simulink model "PistonEngineTestbed"  (R2026a)
settings: Solver=VariableStepAuto  StopTime=0.2  AbsTol=1e-3  EnableMultiTasking=on
libraries: fl_lib x18, nesl_utility x5, sdl_lib x3
CloseFcn:
  | try,close(h1_PistonEngineTestbed),end
  | clear h1_PistonEngineTestbed
  | 
  | 
  | clear simlog_PistonEngineTestbed
Description:
  | Piston Engine Testbed
settings Model: FPTRunName=Active  ExtModeAutoUpdateStatusClock=off  Creator=The MathWorks, Inc.  LastModifiedBy=The MathWorks, Inc.
settings SolverCC: ZcThreshold=0
settings DataIOCC: SignalLoggingName=logsout_PistonEngineTestbed
settings OptimizationCC: InitFltsAndDblsToZero=on  BufferReusableBoundary=off
settings DebuggingCC: SaveWithParameterizedLinksMsg=none  SignalResolutionControl=TryResolveAllWithWarning  MultiTaskDSMMsg=warning  MultiTaskCondExecSysMsg=none  SigSpecEnsureSampleTimeMsg=none  BusObjectLabelMismatch=none  PregeneratedLibrarySubsystemCodeDiagnostic=none
settings HardwareCC: ProdHWDeviceType=32-bit Generic  TargetBitPerPointer=64.0  TargetBitPerSizeT=64.0  TargetBitPerPtrDiffT=64.0  TargetLongLongMode=on  TargetIntDivRoundTo=Zero  TargetEndianess=LittleEndian  TargetWordSize=64.0  TargetHWDeviceType=MATLAB Host  ProdEqTarget=off
settings GRTTargetCC: CombineOutputUpdateFcns=off  GRTInterface=on
settings SimscapeCC: SimscapeNominalValues="[{\"value\":\"1\",\"unit\":\"A\"},{\"value\":\"1\",\"unit\":\"bar\"},{\"value\":\"1\",\"unit\":\"cm^2\"},{\"value\":\"1\",\"unit\":\"cm^3/s\"},{\"value\":\"1\",\"unit\":\"kJ/kg\"},{\"value\":\"1\",\"unit\":\"kW\"},{\"value\":\"1\",\"unit\":\"l\"},{\"value\":\"1\",\"unit\":\"N\"},{\"value\":\"1\",\"unit\":\"N*m\"},{\"value\":\"1\",\"unit\":\"V\"}]"  SimscapeLogSimulationStatistics=on  SimscapeLogName=simlog_PistonEngineTestbed  SimscapeLogDataHistory=5000.0

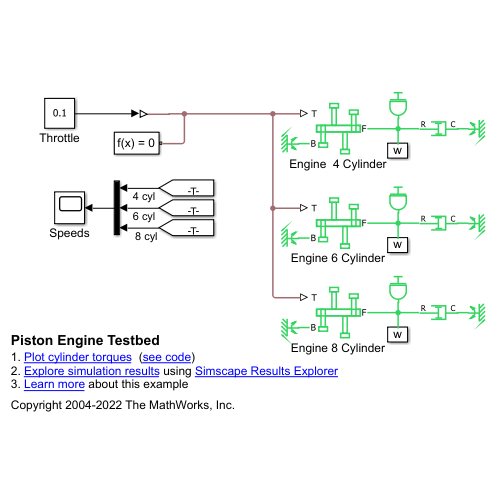
[thumbnail: Simulink's stored preview of the top-level diagram]
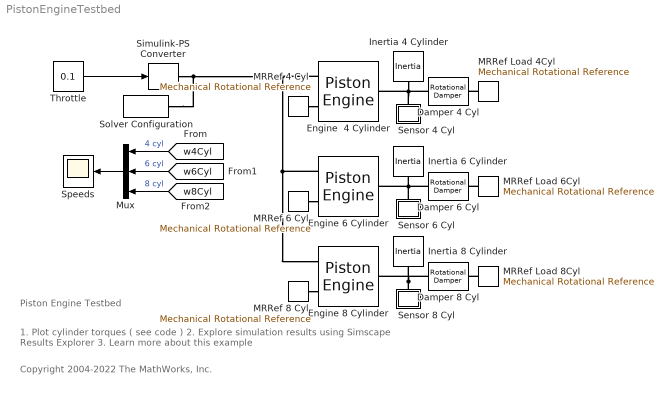
== system PistonEngineTestbed ==
  note: Piston Engine Testbed
  note: 1. Plot cylinder torques ( see code )
      | 2. Explore simulation results using Simscape Results Explorer
      | 3. Learn more about this example
  note: Copyright 2004-2022 The MathWorks, Inc.
  Damper 4 Cyl : fl_lib/Mechanical/Rotational Elements/Rotational Damper  D=0.0885 N*m/(rad/s)  w_specify=off  w_priority=None  w=0 rad/s  w_nominal_specify=off  w_nominal_value=1  w_nominal_unit=rad/s  t_specify=off  t_priority=None  t=0 N*m  t_nominal_specify=off  t_nominal_value=1  t_nominal_unit=N*m
  Damper 6 Cyl : fl_lib/Mechanical/Rotational Elements/Rotational Damper  D=0.0885 N*m/(rad/s)  w_specify=off  w_priority=None  w=0 rad/s  w_nominal_specify=off  w_nominal_value=1  w_nominal_unit=rad/s  t_specify=off  t_priority=None  t=0 N*m  t_nominal_specify=off  t_nominal_value=1  t_nominal_unit=N*m
  Damper 8 Cyl : fl_lib/Mechanical/Rotational Elements/Rotational Damper  D=0.0885 N*m/(rad/s)  w_specify=off  w_priority=None  w=0 rad/s  w_nominal_specify=off  w_nominal_value=1  w_nominal_unit=rad/s  t_specify=off  t_priority=None  t=0 N*m  t_nominal_specify=off  t_nominal_value=1  t_nominal_unit=N*m
  Engine  4 Cylinder : sdl_lib/Engines & Motors/Piston Engine  piston_num=4  theta_offset_vector=[0.0, 180.0, 360.0, -180.0] deg  bore=.10 m  stroke=.06 m  rod=.1 m  stroke_num=4  parameterization=1  angle_vector=[-360.0, -90.0, -30.0, 10.0, 30.0, 90.0, 160.0, 360.0] deg  throttle_vector=[0.0, 0.3, 0.8, 1.0]  velocity_vector=[0.0, 1000.0, 6000.0] rpm  pressure_vector=[0.0, 3.0, 20.0, 50.0, 20.0, 10.0, 8.0, 0.0] bar  pressure_matrix=[0.0, 0.0, 0.0, 0.0; 0.0, 0.9, 2.4, 3.0; 0.0, 6.0, 16.0, 20.0; 0.0, 15.0, 40.0, 50.0; 0.0, 6.0, 16.0, 20.0; 0.0, 3.0, 8.0, 10.0; 0.0, 2.4, 6.4, 8.0; 0.0, 0.0, 0.0, 0.0] bar  pressure_matrix_3D=cat(3, [0.0, 0.0, 0.0, 0.0; 0.0, 0.9, 2.4, 3.0; 0.0, 6.0, 16.0, 20.0; 0.0, 15.0, 40.0, 50.0; 0.0, 6.0, 16.0, 20.0; 0.0, 3.0, 8.0, 10.0; 0.0, 2.4, 6.4, 8.0; 0.0, 0.0, 0.0, 0.0], [0.0, 0.0, 0.0, 0.0; 0.0, 0.9, 2.4, 3.0; 0.0, 6.0, 16.0, 20.0; 0.0, 15.0, 40.0, 50.0; 0.0, 6.0, 16.0, 20.0; 0.0, 3.0, 8.0, 10.0; 0.0, 2.4, 6.4, 8.0; 0.0, 0.0, 0.0, 0.0], [0.0, 0.0, 0.0, 0.0; 0.0, 0.9, 2.4, 3.0; 0.0, 6.0, 16.0, 20.0; 0.0, 15.0, 40.0, 50.0; 0.0, 6.0, 16.0, 20.0; 0.0, 3.0, 8.0, 10.0; 0.0, 2.4, 6.4, 8.0; 0.0, 0.0, 0.0, 0.0]) bar  shaft_dynamics=0  stiffness=1e6 N*m/rad  damping=1000 N*m/(rad/s)  inertia=.02 kg*m^2  initial_deflection=0 deg  initial_velocity=0 rpm  mu_visc=[0.0, 0.01] N*m/(rad/s)  theta_init=0 deg  fc_model=sdl.enum.fuel_consumption_model.FuelOff  fc_per_rev=25 mg/rev  fc_w_tab=[1000, 2000, 3000, 4000, 5000, 6000] rpm  fc_trq_tab=[0, 80, 160, 200, 240, 320, 360, 400] N*m  fc_tab=[.5, .9, 1.4, 1.6, 1.9, 2.7, 3.4, 4.4; 1, 1.7, 2.7, 3.1, 3.6, 5, 6, 7.4; 1.4, 2.7, 4, 4.8, 5.6, 7.5, 8.5, 10.5; 2, 3.6, 5.8, 6.7, 8, 10.4, 11.7, 13.3; 2.5, 4.8, 7.9, 9.4, 10.8, 14, 16.2, 18.6; 3.1, 6, 10.3, 11.9, 13.8, 18.4, 22, 26.5] g/s  bmep_tab=[0, 250, 500, 625, 750, 1000, 1150, 1250] kPa  bsfc_tab=[410, 380, 300, 280, 270, 290, 320, 380; 410, 370, 290, 270, 260, 270, 285, 320; 415, 380, 290, 275, 265, 270, 270, 300; 420, 390, 310, 290, 285, 280, 280, 285; 430, 410, 340, 320, 310, 300, 310, 320; 450, 430, 370, 340, 330, 330, 350, 380] g/hr/kW  fc_interp_method=simscape.enum.interpolation.linear
  Engine 6 Cylinder : sdl_lib/Engines & Motors/Piston Engine  piston_num=6  theta_offset_vector=[0.0, 120.0, 240.0, 360.0, -240.0, -120.0] deg  bore=.10 m  stroke=.06 m  rod=.1 m  stroke_num=4  parameterization=1  angle_vector=[-360.0, -90.0, -30.0, 10.0, 30.0, 90.0, 160.0, 360.0] deg  throttle_vector=[0.0, 0.3, 0.8, 1.0]  velocity_vector=[0.0, 1000.0, 6000.0] rpm  pressure_vector=[0.0, 3.0, 20.0, 50.0, 20.0, 10.0, 8.0, 0.0]*4/6 bar  pressure_matrix=[0.0, 0.0, 0.0, 0.0; 0.0, 0.9, 2.4, 3.0; 0.0, 6.0, 16.0, 20.0; 0.0, 15.0, 40.0, 50.0; 0.0, 6.0, 16.0, 20.0; 0.0, 3.0, 8.0, 10.0; 0.0, 2.4, 6.4, 8.0; 0.0, 0.0, 0.0, 0.0]*4/6 bar  pressure_matrix_3D=cat(3, [0.0, 0.0, 0.0, 0.0; 0.0, 0.9, 2.4, 3.0; 0.0, 6.0, 16.0, 20.0; 0.0, 15.0, 40.0, 50.0; 0.0, 6.0, 16.0, 20.0; 0.0, 3.0, 8.0, 10.0; 0.0, 2.4, 6.4, 8.0; 0.0, 0.0, 0.0, 0.0], [0.0, 0.0, 0.0, 0.0; 0.0, 0.9, 2.4, 3.0; 0.0, 6.0, 16.0, 20.0; 0.0, 15.0, 40.0, 50.0; 0.0, 6.0, 16.0, 20.0; 0.0, 3.0, 8.0, 10.0; 0.0, 2.4, 6.4, 8.0; 0.0, 0.0, 0.0, 0.0], [0.0, 0.0, 0.0, 0.0; 0.0, 0.9, 2.4, 3.0; 0.0, 6.0, 16.0, 20.0; 0.0, 15.0, 40.0, 50.0; 0.0, 6.0, 16.0, 20.0; 0.0, 3.0, 8.0, 10.0; 0.0, 2.4, 6.4, 8.0; 0.0, 0.0, 0.0, 0.0])*4/6 bar  shaft_dynamics=0  stiffness=1e6 N*m/rad  damping=1000 N*m/(rad/s)  inertia=.02 kg*m^2  initial_deflection=0 deg  initial_velocity=0 rpm  mu_visc=[0.0, 0.01] N*m/(rad/s)  theta_init=0 deg  fc_model=sdl.enum.fuel_consumption_model.FuelOff  fc_per_rev=25 mg/rev  fc_w_tab=[1000, 2000, 3000, 4000, 5000, 6000] rpm  fc_trq_tab=[0, 80, 160, 200, 240, 320, 360, 400] N*m  fc_tab=[.5, .9, 1.4, 1.6, 1.9, 2.7, 3.4, 4.4; 1, 1.7, 2.7, 3.1, 3.6, 5, 6, 7.4; 1.4, 2.7, 4, 4.8, 5.6, 7.5, 8.5, 10.5; 2, 3.6, 5.8, 6.7, 8, 10.4, 11.7, 13.3; 2.5, 4.8, 7.9, 9.4, 10.8, 14, 16.2, 18.6; 3.1, 6, 10.3, 11.9, 13.8, 18.4, 22, 26.5] g/s  bmep_tab=[0, 250, 500, 625, 750, 1000, 1150, 1250] kPa  bsfc_tab=[410, 380, 300, 280, 270, 290, 320, 380; 410, 370, 290, 270, 260, 270, 285, 320; 415, 380, 290, 275, 265, 270, 270, 300; 420, 390, 310, 290, 285, 280, 280, 285; 430, 410, 340, 320, 310, 300, 310, 320; 450, 430, 370, 340, 330, 330, 350, 380] g/hr/kW  fc_interp_method=simscape.enum.interpolation.linear
  Engine 8 Cylinder : sdl_lib/Engines & Motors/Piston Engine  piston_num=8  theta_offset_vector=[0.0, 90.0, 180.0, 270.0, 360.0, -90.0, -180.0, -270.0] deg  bore=.10 m  stroke=.06 m  rod=.1 m  stroke_num=4  parameterization=1  angle_vector=[-360.0, -90.0, -30.0, 10.0, 30.0, 90.0, 160.0, 360.0] deg  throttle_vector=[0.0, 0.3, 0.8, 1.0]  velocity_vector=[0.0, 1000.0, 6000.0] rpm  pressure_vector=[0.0, 3.0, 20.0, 50.0, 20.0, 10.0, 8.0, 0.0]*4/8 bar  pressure_matrix=[0.0, 0.0, 0.0, 0.0; 0.0, 0.9, 2.4, 3.0; 0.0, 6.0, 16.0, 20.0; 0.0, 15.0, 40.0, 50.0; 0.0, 6.0, 16.0, 20.0; 0.0, 3.0, 8.0, 10.0; 0.0, 2.4, 6.4, 8.0; 0.0, 0.0, 0.0, 0.0]*4/8 bar  pressure_matrix_3D=cat(3, [0.0, 0.0, 0.0, 0.0; 0.0, 0.9, 2.4, 3.0; 0.0, 6.0, 16.0, 20.0; 0.0, 15.0, 40.0, 50.0; 0.0, 6.0, 16.0, 20.0; 0.0, 3.0, 8.0, 10.0; 0.0, 2.4, 6.4, 8.0; 0.0, 0.0, 0.0, 0.0], [0.0, 0.0, 0.0, 0.0; 0.0, 0.9, 2.4, 3.0; 0.0, 6.0, 16.0, 20.0; 0.0, 15.0, 40.0, 50.0; 0.0, 6.0, 16.0, 20.0; 0.0, 3.0, 8.0, 10.0; 0.0, 2.4, 6.4, 8.0; 0.0, 0.0, 0.0, 0.0], [0.0, 0.0, 0.0, 0.0; 0.0, 0.9, 2.4, 3.0; 0.0, 6.0, 16.0, 20.0; 0.0, 15.0, 40.0, 50.0; 0.0, 6.0, 16.0, 20.0; 0.0, 3.0, 8.0, 10.0; 0.0, 2.4, 6.4, 8.0; 0.0, 0.0, 0.0, 0.0])*4/8 bar  shaft_dynamics=0  stiffness=1e6 N*m/rad  damping=1000 N*m/(rad/s)  inertia=.02 kg*m^2  initial_deflection=0 deg  initial_velocity=0 rpm  mu_visc=[0.0, 0.01] N*m/(rad/s)  theta_init=0 deg  fc_model=sdl.enum.fuel_consumption_model.FuelOff  fc_per_rev=25 mg/rev  fc_w_tab=[1000, 2000, 3000, 4000, 5000, 6000] rpm  fc_trq_tab=[0, 80, 160, 200, 240, 320, 360, 400] N*m  fc_tab=[.5, .9, 1.4, 1.6, 1.9, 2.7, 3.4, 4.4; 1, 1.7, 2.7, 3.1, 3.6, 5, 6, 7.4; 1.4, 2.7, 4, 4.8, 5.6, 7.5, 8.5, 10.5; 2, 3.6, 5.8, 6.7, 8, 10.4, 11.7, 13.3; 2.5, 4.8, 7.9, 9.4, 10.8, 14, 16.2, 18.6; 3.1, 6, 10.3, 11.9, 13.8, 18.4, 22, 26.5] g/s  bmep_tab=[0, 250, 500, 625, 750, 1000, 1150, 1250] kPa  bsfc_tab=[410, 380, 300, 280, 270, 290, 320, 380; 410, 370, 290, 270, 260, 270, 285, 320; 415, 380, 290, 275, 265, 270, 270, 300; 420, 390, 310, 290, 285, 280, 280, 285; 430, 410, 340, 320, 310, 300, 310, 320; 450, 430, 370, 340, 330, 330, 350, 380] g/hr/kW  fc_interp_method=simscape.enum.interpolation.linear
  Inertia 4 Cylinder : fl_lib/Mechanical/Rotational Elements/Inertia  inertia=1 kg*m^2  num_ports=foundation.enum.numPorts2.one  w_specify=on  w_priority=High  w=800 rpm  w_nominal_specify=off  w_nominal_value=1  w_nominal_unit=rad/s  t_specify=off  t_priority=None  t=0 N*m  t_nominal_specify=off  t_nominal_value=1  t_nominal_unit=N*m
  Inertia 6 Cylinder : fl_lib/Mechanical/Rotational Elements/Inertia  inertia=1 kg*m^2  num_ports=foundation.enum.numPorts2.one  w_specify=on  w_priority=High  w=800 rpm  w_nominal_specify=off  w_nominal_value=1  w_nominal_unit=rad/s  t_specify=off  t_priority=None  t=0 N*m  t_nominal_specify=off  t_nominal_value=1  t_nominal_unit=N*m
  Inertia 8 Cylinder : fl_lib/Mechanical/Rotational Elements/Inertia  inertia=1 kg*m^2  num_ports=foundation.enum.numPorts2.one  w_specify=on  w_priority=High  w=800 rpm  w_nominal_specify=off  w_nominal_value=1  w_nominal_unit=rad/s  t_specify=off  t_priority=None  t=0 N*m  t_nominal_specify=off  t_nominal_value=1  t_nominal_unit=N*m
  MRRef Load 8Cyl : fl_lib/Mechanical/Rotational Elements/Mechanical Rotational Reference
  MRRef 4 Cyl : fl_lib/Mechanical/Rotational Elements/Mechanical Rotational Reference
  MRRef 6 Cyl : fl_lib/Mechanical/Rotational Elements/Mechanical Rotational Reference
  MRRef 8 Cyl : fl_lib/Mechanical/Rotational Elements/Mechanical Rotational Reference
  MRRef Load 4Cyl : fl_lib/Mechanical/Rotational Elements/Mechanical Rotational Reference
  MRRef Load 6Cyl : fl_lib/Mechanical/Rotational Elements/Mechanical Rotational Reference
  Mux : Mux  Inputs=3
  Sensor 4 Cyl : Subsystem
      mask Display: disp('w');
  Sensor 6 Cyl : Subsystem
      mask Display: disp('w');
  Sensor 8 Cyl : Subsystem
      mask Display: disp('w');
  Simulink-PS Converter : nesl_utility/Simulink-PS Converter  PhysicalDomain=network_engine_domain  SubClassName=ps_input  LeftPortType=input  RightPortType=output  PseudoPeriodic=off  Frequencies=[]  NoiseDistribution=none  NoiseParameters=[]  Unit=1  AffineConversion=off  FilteringAndDerivatives=zero  SimscapeFilterOrder=1  InputFilterTimeConstant=0.001  UdotUserProvided=1
  Solver Configuration : nesl_utility/Solver Configuration  PhysicalDomain=network_engine_domain  SubClassName=solver  LeftPortType=input  RightPortType=generic  Tones=[]  Harmonics=[]  SimulateNoise=off  Profile=off  UseLocalSampling=off  EnableSwitchedLinearOptims=on  FrequencyDomain=off  UseCCode=off  RelTol=0.001  AbsTol=1e-06  MinStep=1e-09  ToWorkspace=off  RevertToSquareIcSolve=off  NumHomotopyIterations=100  PhasorMode=off  PhasorModeNumHarmonics=1  ConsistencySolver=NEWTON_XTOL_AFTER_FTOL  CanonicalOrdering=UNORDERED  OptimizeIntermediates=UNOPTIMIZED  IndexReductionMethod=DerivativeReplacement  DoDC=off  ResidualTolerance=1e-9  ConsistencyTolSource=GLOBAL  ConsistencyAbsTol=0.001  ConsistencyRelTol=0.001  ConsistencyTolFactor=0.001  UseLocalSolver=off  LocalSolverChoice=NE_PARTITIONING_ADVANCER  ResolveIndetEquations=on  FunctionEvalNumThread=1  LocalSolverSampleTime=0.001  DoFixedCost=off  MaxNonlinIter=3  MaxModeIter=2  ComputeImpulses=off  ImpulseIterations=2  LinearAlgebra=auto  LinearAlgebraNumThread=0  EquationFormulation=NE_TIME_EF  DelaysMemoryBudget=1024  AutomaticFiltering=on  FilteringTimeConstant=0.001  PartitionStorageMethod=EXHAUSTIVE  PartitionMemoryBudget=1024  PartitionMethod=ROBUST  MultibodyUseLocalSolver=off  MultibodyLocalSolverChoice=ODE1  MultibodyLocalSolverSampleTime=0.001
  Speeds : Scope
      settings: Title=Engine Speed  ActiveDisplayYMinimum=799.61316  ActiveDisplayYMaximum=802.91945
  Throttle : Constant  Value=0.1
  wires:
  Throttle/1 -> Simulink-PS Converter/1
  [w8Cyl] -> Mux/3  "8 cyl"
  Mux/1 -> Speeds/1
  [w4Cyl] -> Mux/1  "4 cyl"
  [w6Cyl] -> Mux/2  "6 cyl"
  connections:
  Simulink-PS Converter/RConn1 -- Solver Configuration/RConn1 -- Engine  4 Cylinder/LConn1 -- Engine 6 Cylinder/LConn1 -- Engine 8 Cylinder/LConn1
  MRRef 8 Cyl/LConn1 -- Engine 8 Cylinder/LConn2
  MRRef 6 Cyl/LConn1 -- Engine 6 Cylinder/LConn2
  MRRef 4 Cyl/LConn1 -- Engine  4 Cylinder/LConn2
  Sensor 4 Cyl/LConn1 -- Damper 4 Cyl/LConn1 -- Inertia 4 Cylinder/LConn1 -- Engine  4 Cylinder/RConn1
  Inertia 8 Cylinder/LConn1 -- Engine 8 Cylinder/RConn1 -- Damper 8 Cyl/LConn1 -- Sensor 8 Cyl/LConn1
  MRRef Load 4Cyl/LConn1 -- Damper 4 Cyl/RConn1
  MRRef Load 6Cyl/LConn1 -- Damper 6 Cyl/RConn1
  Sensor 6 Cyl/LConn1 -- Damper 6 Cyl/LConn1 -- Inertia 6 Cylinder/LConn1 -- Engine 6 Cylinder/RConn1
  MRRef Load 8Cyl/LConn1 -- Damper 8 Cyl/RConn1

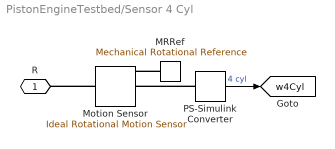
== system PistonEngineTestbed/Sensor 4 Cyl ==
  MRRef : fl_lib/Mechanical/Rotational Elements/Mechanical Rotational Reference
  Motion Sensor : fl_lib/Mechanical/Mechanical Sensors/Ideal Rotational Motion Sensor  reference=foundation.enum.MeasurementReference.difference  acceleration_port=false  velocity_port=true  position_port=true  wrap_angle=simscape.enum.onoff.off  offset=0 rad
  PS-Simulink Converter : nesl_utility/PS-Simulink Converter  PhysicalDomain=network_engine_domain  SubClassName=ps_output  LeftPortType=input  RightPortType=output  PseudoPeriodic=off  Frequencies=[]  VectorFormat=1-D array  Unit=rpm  AffineConversion=off
  R : PMIOPort  Side=Left
  tag scope: w4Cyl=global
  wires:
  PS-Simulink Converter/1 -> [w4Cyl]  "4 cyl"
  connections:
  Motion Sensor/LConn1 -- R/RConn1
  PS-Simulink Converter/LConn1 -- Motion Sensor/RConn2
  MRRef/LConn1 -- Motion Sensor/RConn1

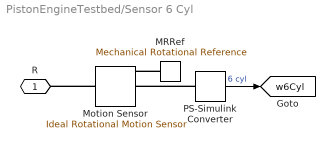
== system PistonEngineTestbed/Sensor 6 Cyl ==
  MRRef : fl_lib/Mechanical/Rotational Elements/Mechanical Rotational Reference
  Motion Sensor : fl_lib/Mechanical/Mechanical Sensors/Ideal Rotational Motion Sensor  reference=foundation.enum.MeasurementReference.difference  acceleration_port=false  velocity_port=true  position_port=true  wrap_angle=simscape.enum.onoff.off  offset=0 rad
  PS-Simulink Converter : nesl_utility/PS-Simulink Converter  PhysicalDomain=network_engine_domain  SubClassName=ps_output  LeftPortType=input  RightPortType=output  PseudoPeriodic=off  Frequencies=[]  VectorFormat=1-D array  Unit=rpm  AffineConversion=off
  R : PMIOPort  Side=Left
  tag scope: w6Cyl=global
  wires:
  PS-Simulink Converter/1 -> [w6Cyl]  "6 cyl"
  connections:
  MRRef/LConn1 -- Motion Sensor/RConn1
  PS-Simulink Converter/LConn1 -- Motion Sensor/RConn2
  Motion Sensor/LConn1 -- R/RConn1

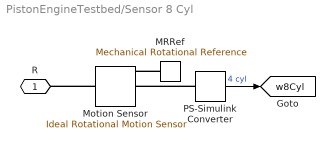
== system PistonEngineTestbed/Sensor 8 Cyl ==
  MRRef : fl_lib/Mechanical/Rotational Elements/Mechanical Rotational Reference
  Motion Sensor : fl_lib/Mechanical/Mechanical Sensors/Ideal Rotational Motion Sensor  reference=foundation.enum.MeasurementReference.difference  acceleration_port=false  velocity_port=true  position_port=true  wrap_angle=simscape.enum.onoff.off  offset=0 rad
  PS-Simulink Converter : nesl_utility/PS-Simulink Converter  PhysicalDomain=network_engine_domain  SubClassName=ps_output  LeftPortType=input  RightPortType=output  PseudoPeriodic=off  Frequencies=[]  VectorFormat=1-D array  Unit=rpm  AffineConversion=off
  R : PMIOPort  Side=Left
  tag scope: w8Cyl=global
  wires:
  PS-Simulink Converter/1 -> [w8Cyl]  "4 cyl"
  connections:
  Motion Sensor/LConn1 -- R/RConn1
  PS-Simulink Converter/LConn1 -- Motion Sensor/RConn2
  MRRef/LConn1 -- Motion Sensor/RConn1
